simulink model "H8_2GDL_Comparacion_Lineal_NoLineal"  (R2022b)
settings: Solver=VariableStepAuto  StartTime=0.0  StopTime=0.1  RelTol=1e-3
InitFcn:
  | load("hems.mat");
  | airgap = hems.Airgap;
  | current = hems.Current;
  | forceV = hems.Force_Vertical;
  | forceH = hems.Force_Horizontal;
  | inductance = hems.Inductance;
  | resistance = hems.Resistance;
  | 
  | m = 200;
  | g = 9.81;
  | Iyy = 26.887;
  | x_lev12 = 0.443;
  | x_lev34 = 0.542;
  | z_max = 0.0225;
  | z_min = 0.01;
  | z_nom = 0.019375;
  | I_max = 50;
  | I_min = -50;
values from neighbouring files (symbols this model uses):
  A2 = argout.a    [linealizacion_2gdl.m]    (also in matrices_lineal_2gdl.mat = [0 0 689.948845287 37.4788996561 0 0 139.394129714 757.14948)
  B2 = argout.b    [linealizacion_2gdl.m]    (also in matrices_lineal_2gdl.mat = [0  0; 0  0; 0.151630617985  -0.185516467151; -0.09202917439)
  C2 = argout.c    [linealizacion_2gdl.m]    (also in matrices_lineal_2gdl.mat = [1 0 0 0 0 1 0 0 0 0 1 0 ... (16 elements, 4x4)])
  D2 = argout.d    [linealizacion_2gdl.m]    (also in matrices_lineal_2gdl.mat = [0  0; 0  0; 0  0; 0  0])
settings Model: Creator=aceao  LastModifiedBy=aceao

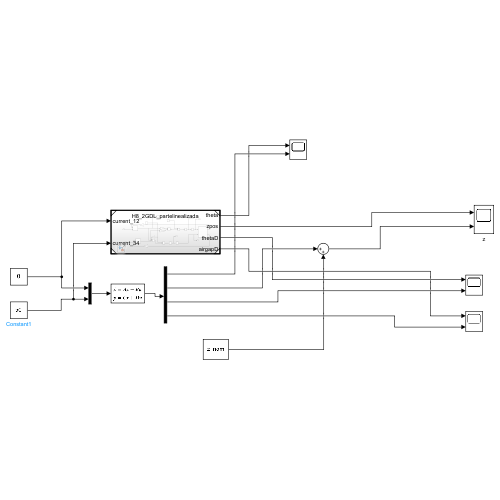
[thumbnail: Simulink's stored preview of the top-level diagram]
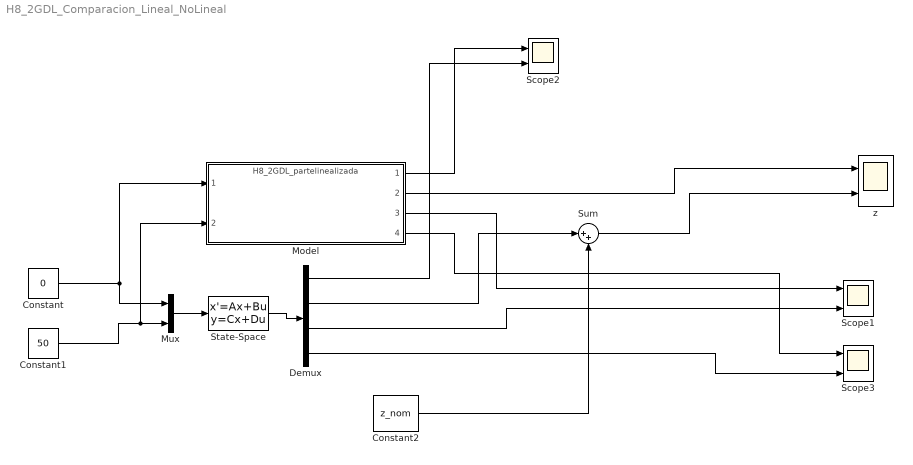
== system H8_2GDL_Comparacion_Lineal_NoLineal ==
  Constant : Constant  Value=0
  Constant1 : Constant  Value=50
  Constant2 : Constant  Value=z_nom
  Demux : Demux
  Model : ModelReference  ModelNameDialog=H8_2GDL_partelinealizada.slx  SimulationMode=Normal  ModelReferenceVersion=1.31
  Mux : Mux  Inputs=2
  Scope1 : Scope  NumInputPorts=2
  Scope2 : Scope  NumInputPorts=2
  Scope3 : Scope  NumInputPorts=2
  State-Space : StateSpace  A=A2  B=B2  C=C2  D=D2  InitialCondition=[0, 0, 0, 0]
  Sum : Sum  Inputs=|++
  z : Scope  NumInputPorts=2
  wires:
  Mux/1 -> State-Space/1
  Constant/1 -> Model/1, Mux/1
  Constant1/1 -> Model/2, Mux/2
  State-Space/1 -> Demux/1
  Model/1 -> Scope2/1
  Demux/1 -> Scope2/2
  Demux/2 -> Sum/1
  Constant2/1 -> Sum/2
  Model/3 -> Scope1/1
  Demux/3 -> Scope1/2
  Demux/4 -> Scope3/2
  Model/4 -> Scope3/1
  Model/2 -> z/1
  Sum/1 -> z/2
